simulink model "DinamicaInversa"  (R2020a)
settings: Solver=VariableStepAuto  StartTime=0.0  StopTime=5  RelTol=1e-3
undefined symbols (not defined in the file or in its folder): din_inv, robot
settings Model: Creator=agroo  LastModifiedBy=agroo

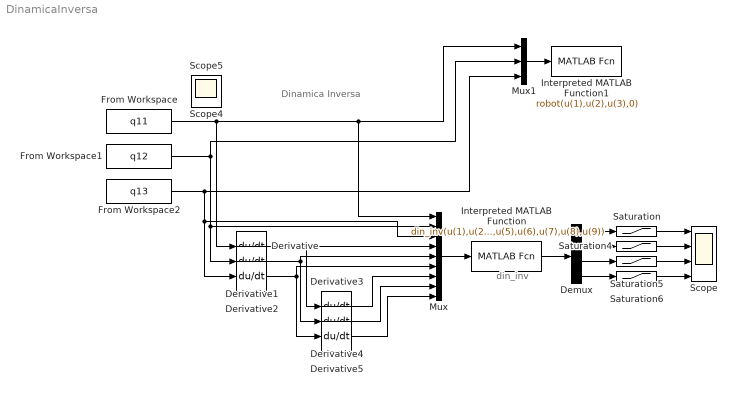
== system DinamicaInversa ==
  note: din_inv
  note: Dinamica Inversa
  Demux : Demux
  Derivative{,1..5} (6 alike) : Derivative
  From Workspace : FromWorkspace  VariableName=q11
  From Workspace1 : FromWorkspace  VariableName=q12
  From Workspace2 : FromWorkspace  VariableName=q13
  Interpreted MATLAB Function : MATLABFcn  MATLABFcn=din_inv(u(1),u(2),u(3),u(4),u(5),u(6),u(7),u(8),u(9))  OutputDimensions=4
  Interpreted MATLAB Function1 : MATLABFcn  MATLABFcn=robot(u(1),u(2),u(3),0)  OutputDimensions=0
  Mux : Mux  Inputs=9
  Mux1 : Mux  Inputs=3
  Saturation : Saturate  UpperLimit=20  LowerLimit=-20
  Saturation4 : Saturate  UpperLimit=25  LowerLimit=-25
  Saturation5 : Saturate  UpperLimit=18  LowerLimit=-18
  Saturation6 : Saturate  UpperLimit=5  LowerLimit=-5
  Scope : Scope  NumInputPorts=4
  Scope4 : Scope
  Scope5 : Scope
  wires:
  Mux/1 -> Interpreted MATLAB Function/1
  From Workspace/1 -> Derivative/1, Mux1/1, Mux/1
  Interpreted MATLAB Function/1 -> Demux/1
  From Workspace2/1 -> Mux1/3, Derivative2/1, Mux/3
  From Workspace1/1 -> Derivative1/1, Mux/2, Mux1/2
  Derivative/1 -> Mux/4, Derivative3/1
  Derivative1/1 -> Derivative4/1, Mux/5
  Derivative2/1 -> Mux/6, Derivative5/1
  Derivative3/1 -> Mux/7
  Derivative4/1 -> Mux/8
  Derivative5/1 -> Mux/9
  Mux1/1 -> Interpreted MATLAB Function1/1
  Demux/1 -> Saturation/1
  Saturation/1 -> Scope/1
  Demux/2 -> Saturation4/1
  Saturation4/1 -> Scope/2
  Demux/3 -> Saturation5/1
  Saturation5/1 -> Scope/3
  Demux/4 -> Saturation6/1
  Saturation6/1 -> Scope/4
